simulink model "haromszereplos"  (Simulink 7.8)
settings: Solver=ode45  StartTime=0.0  StopTime=50.0  RelTol=1e-3
libraries: simulink x1
settings Model: Creator=valaki  LastModifiedBy=valaki

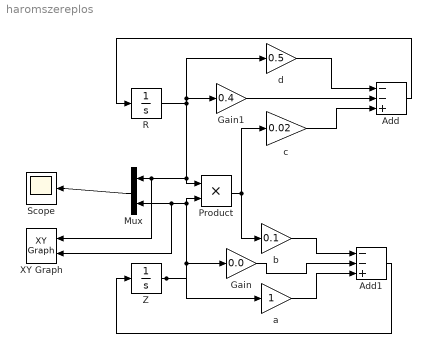
== system haromszereplos ==
  Add : Sum  Inputs=--+
  Add1 : Sum  Inputs=--+
  Gain : Gain  Gain=0.0
  Gain1 : Gain  Gain=0.4
  Mux : Mux  Inputs=2
  Product : Product  RndMeth=Zero
  R : Integrator  InitialCondition=13
  Scope : Scope
  XY Graph : simulink/Sinks/XY Graph  xmin=0  xmax=30  ymin=0  ymax=60  st=-1
  Z : Integrator  InitialCondition=25
  a : Gain
  b : Gain  Gain=0.1
  c : Gain  Gain=0.02
  d : Gain  Gain=0.5
  wires:
  d/1 -> Add/1
  R/1 -> Product/1, Mux/1, XY Graph/1, d/1, Gain1/1
  Product/1 -> c/1, b/1
  Z/1 -> a/1, Product/2, Mux/2, XY Graph/2, Gain/1
  b/1 -> Add1/1
  Add/1 -> R/1
  Add1/1 -> Z/1
  Mux/1 -> Scope/1
  a/1 -> Add1/3
  Gain/1 -> Add1/2
  c/1 -> Add/3
  Gain1/1 -> Add/2
